simulink model "passive"  (R2021a)
settings: Solver=VariableStepAuto  StartTime=0.0  StopTime=1  RelTol=1e-3
undefined symbols (not defined in the file): Ion, Lithium
libraries: spsSeriesRLCBranchLib x4, spsBatteryLib x3, spsMosfetLib x3, spsIdealSwitchLib x2, spsDCVoltageSourceLib x1, spspowerguiLib x1
settings Model: Creator=sampa  LastModifiedBy=sampa

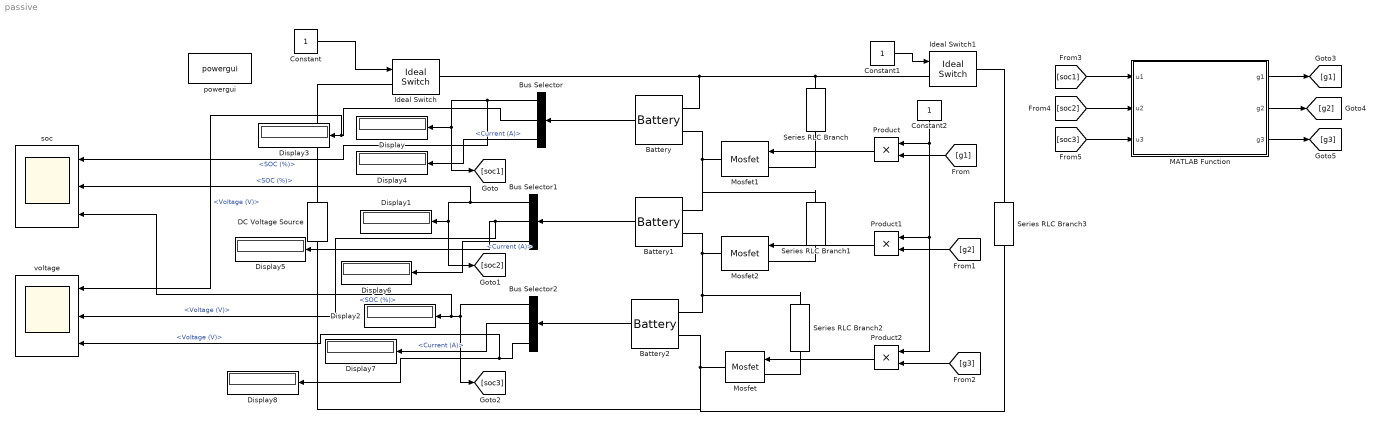
== system passive ==
  Battery : spsBatteryLib/Battery  BatType=Lithium-Ion  ShowTempParam=off  ThermalPreset=no  ShowAgeParam=off  NomV=7.2  NomQ=5.7  SOC=50  Batt_Tr=30  PresetModel=on  MaxQ=5.7  MinV=5.4  FullV=8.3807  Dis_rate=2.4783  R=0.012632  Normal_OP=5.1548  expZone="[7.7788     0.28004]"  current=[6.5 13 32.5]  Units=Time  Tci=20  NomT=20  T2=-30  MaxQ2=4.8  FullV2=7.1  Normal_OP2=5.655  expZone2="[6.58           1]"  Rca=0.6  ti=2000  Dp=0  Neq0=0  Tsim=1e6  Ta1=25  Qeol=5.4*0.9  Reol=0.013333*1.2  Char_age=[2.3478, 3]  Dis_age=[2.3478, 10]  N1=1500  N2=10500  N3=1000  N4=1400  Ta2=45  N5=950
  Battery1 : spsBatteryLib/Battery  BatType=Lithium-Ion  ShowTempParam=off  ThermalPreset=no  ShowAgeParam=off  NomV=7.2  NomQ=5.7  SOC=70  Batt_Tr=30  PresetModel=on  MaxQ=5.7  MinV=5.4  FullV=8.3807  Dis_rate=2.4783  R=0.012632  Normal_OP=5.1548  expZone="[7.7788     0.28004]"  current=[6.5 13 32.5]  Units=Time  Tci=20  NomT=20  T2=-30  MaxQ2=4.8  FullV2=7.1  Normal_OP2=5.655  expZone2="[6.58           1]"  Rca=0.6  ti=2000  Dp=0  Neq0=0  Tsim=1e6  Ta1=25  Qeol=5.4*0.9  Reol=0.013333*1.2  Char_age=[2.3478, 3]  Dis_age=[2.3478, 10]  N1=1500  N2=10500  N3=1000  N4=1400  Ta2=45  N5=950
  Battery2 : spsBatteryLib/Battery  BatType=Lithium-Ion  ShowTempParam=off  ThermalPreset=no  ShowAgeParam=off  NomV=7.2  NomQ=5.7  SOC=100  Batt_Tr=30  PresetModel=on  MaxQ=5.7  MinV=5.4  FullV=8.3807  Dis_rate=2.4783  R=0.012632  Normal_OP=5.1548  expZone="[7.7788     0.28004]"  current=[6.5 13 32.5]  Units=Time  Tci=20  NomT=20  T2=-30  MaxQ2=4.8  FullV2=7.1  Normal_OP2=5.655  expZone2="[6.58           1]"  Rca=0.6  ti=2000  Dp=0  Neq0=0  Tsim=1e6  Ta1=25  Qeol=5.4*0.9  Reol=0.013333*1.2  Char_age=[2.3478, 3]  Dis_age=[2.3478, 10]  N1=1500  N2=10500  N3=1000  N4=1400  Ta2=45  N5=950
  Bus Selector : BusSelector  OutputSignals=SOC (%),Voltage (V),Current (A)
  Bus Selector1 : BusSelector  OutputSignals=SOC (%),Voltage (V),Current (A)
  Bus Selector2 : BusSelector  OutputSignals=SOC (%),Current (A),Voltage (V)
  Constant : Constant
  Constant1 : Constant
  Constant2 : Constant
  DC Voltage Source : spsDCVoltageSourceLib/DC Voltage Source  Amplitude=120  Measurements=None
  Display{,1..8} (9 alike) : Display
  Ideal Switch : spsIdealSwitchLib/Ideal Switch  Ron=0.001  Lon=0  IC=0  Rs=1e5  Cs=inf  Measurements=off
  Ideal Switch1 : spsIdealSwitchLib/Ideal Switch  Ron=0.001  Lon=0  IC=0  Rs=1e5  Cs=inf  Measurements=off
  MATLAB Function : MATLAB Function  TreatAsAtomicUnit=on
  Mosfet : spsMosfetLib/Mosfet  Ron=0.1  Lon=0  Rd=0.01  Vfd=0  IC=0  Rs=1e5  Cs=inf  Measurements=off
  Mosfet1 : spsMosfetLib/Mosfet  Ron=0.1  Lon=0  Rd=0.01  Vfd=0  IC=0  Rs=1e5  Cs=inf  Measurements=off
  Mosfet2 : spsMosfetLib/Mosfet  Ron=0.1  Lon=0  Rd=0.01  Vfd=0  IC=0  Rs=1e5  Cs=inf  Measurements=off
  Product : Product
  Product1 : Product
  Product2 : Product
  Series RLC Branch{,1..3} (4 alike) : spsSeriesRLCBranchLib/Series RLC Branch  LConnTagsString=__new0  RConnTagsString=__new0  BranchType=R  Resistance=1  Inductance=1e-3  SetiL0=off  InitialCurrent=0  Capacitance=1e-6  Setx0=off  InitialVoltage=0  Measurements=None
  powergui : spspowerguiLib/powergui  Priority=1  SimulationMode=Continuous  SampleTime=50e-6  frequency=60  Iterations=50  frequencyindice=0  Pbase=100e6  ErrMax=1e-4  UnitsV=kV  UnitsW=MW  buscounter=0  FunctionMessages=off  echomessages=off  EnableUseOfTLC=off  CurrentSourceSwitches=off  DisableSnubberDevices=off  DisableRonSwitches=off  DisableVfSwitches=off  DisplayEquations=off  AutomaticDiscreteSolvers=off  SolverType=Tustin/Backward Euler (TBE)  Interpol=off  ExternalGateDelay=off  methode=off  Ts=100  x0status=blocks  SPID=on  SwTol=0  HookPort=off  NonlinearTolerance=1e-4  nMaxIteration=100  ContinueOnMaxIteration=off  RestoreLinks=warning  ResistiveCurrentMeasurement=off  Frange=[0:2:500]  Ylog=off  Xlog=on  ShowGrid=off  save=off  variable=ZData  structure=0  ZoomFFT=off  StartTime=0.0  cycles=1  DisplayStyle=1  fundamental=60  FreqAxis=off  MaxFrequency=1000  frequencyindicesteady=1  RmsSteady=1  display=off
  soc : Scope  NumInputPorts=3
  voltage : Scope  NumInputPorts=3
  wires:
  Constant/1 -> Ideal Switch/1
  Constant1/1 -> Ideal Switch1/1
  Battery/1 -> Bus Selector/1
  Bus Selector/1 -> soc/1, [soc1], Display/1  "<SOC (%)>"
  Battery2/1 -> Bus Selector2/1
  Bus Selector2/1 -> [soc3], soc/3, Display2/1  "<SOC (%)>"
  Battery1/1 -> Bus Selector1/1
  Bus Selector1/1 -> soc/2, [soc2], Display1/1  "<SOC (%)>"
  Product/1 -> Mosfet1/1
  Product1/1 -> Mosfet2/1
  Product2/1 -> Mosfet/1
  Constant2/1 -> Product/1, Product1/1, Product2/1
  [g1] -> Product/2
  [g3] -> Product2/2
  [g2] -> Product1/2
  [soc1] -> MATLAB Function/1(u1)
  [soc2] -> MATLAB Function/2(u2)
  [soc3] -> MATLAB Function/3(u3)
  MATLAB Function/1(g1) -> [g1]
  MATLAB Function/2(g2) -> [g2]
  MATLAB Function/3(g3) -> [g3]
  Bus Selector/3 -> Display4/1  "<Current (A)>"
  Bus Selector/2 -> voltage/1, Display3/1  "<Voltage (V)>"
  Bus Selector1/2 -> voltage/2, Display5/1  "<Voltage (V)>"
  Bus Selector1/3 -> Display6/1  "<Current (A)>"
  Bus Selector2/2 -> Display7/1  "<Current (A)>"
  Bus Selector2/3 -> voltage/3, Display8/1  "<Voltage (V)>"
  connections:
  Series RLC Branch/LConn1 -- Battery/LConn1 -- Ideal Switch/RConn1 -- Ideal Switch1/LConn1
  Mosfet/LConn1 -- Series RLC Branch2/RConn1
  Mosfet/RConn1 -- DC Voltage Source/LConn1 -- Series RLC Branch3/RConn1 -- Battery2/LConn2
  Mosfet2/LConn1 -- Series RLC Branch1/RConn1
  Battery2/LConn1 -- Series RLC Branch2/LConn1 -- Battery1/LConn2 -- Mosfet2/RConn1
  Mosfet1/LConn1 -- Series RLC Branch/RConn1
  Mosfet1/RConn1 -- Series RLC Branch1/LConn1 -- Battery1/LConn1 -- Battery/LConn2
  Ideal Switch1/RConn1 -- Series RLC Branch3/LConn1
  Ideal Switch/LConn1 -- DC Voltage Source/RConn1

== matlab function passive/MATLAB Function ==
  data: u1 input; g1 output; u2 input; u3 input; g2 output; g3 output
 function [g1,g2,g3] = fcn(u1,u2,u3)

u1 = u1*1000;
u2 = u2*1000;
u3 = u3*1000;

u1 = int32(u1);
u2 = int32(u2);
u3 = int32(u3);

if u1>u2||u1>u3
    g1 = 1;
else g1 = 0;
end
 if u2>u1||u2>u3
     g2 = 1;
 else g2 = 0;
 end
     if u3>u1||u3>u2
         g3 = 1;
     else g3 = 0;
     end
